simulink subsystem "InverseKinematics"  (R2024b)
settings: Solver=VariableStepAuto  StartTime=0.0  StopTime=10.0  RelTol=1e-3
undefined symbols (not defined in the file or in its folder): l, r
settings Model: Creator=Matthew  LastModifiedBy=Matthew

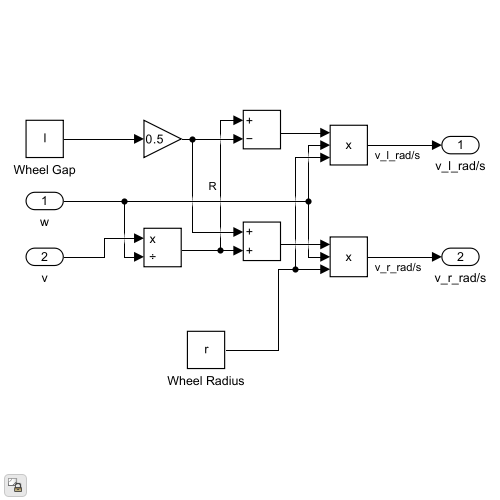
[thumbnail: Simulink's stored preview of the top-level diagram]
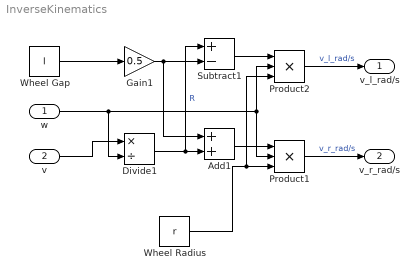
== system InverseKinematics ==
  w : Inport
  v : Inport  Port=2
  Add1 : Sum
  Divide1 : Product  Inputs=*/
  Gain1 : Gain  Gain=0.5
  Product1 : Product  Inputs=3
  Product2 : Product  Inputs=3
  Subtract1 : Sum  Inputs=+-
  Wheel Gap : Constant  Value=l
  Wheel Radius : Constant  Value=r
  v_l_rad/s : Outport
  v_r_rad/s : Outport  Port=2
  wires:
  Wheel Gap/1 -> Gain1/1
  w/1 -> Product2/2, Product1/2, Divide1/2
  Divide1/1 -> Subtract1/1, Add1/2  "R"
  Gain1/1 -> Subtract1/2, Add1/1
  Subtract1/1 -> Product2/1
  Add1/1 -> Product1/1
  Product1/1 -> v_r_rad/s/1  "v_r_rad/s"
  Product2/1 -> v_l_rad/s/1  "v_l_rad/s"
  Wheel Radius/1 -> Product2/3, Product1/3
  v/1 -> Divide1/1
